simulink model "x11_foc_iden_flux"  (R2023b)
settings: Solver=VariableStepAuto  StartTime=0.0  StopTime=0.5  RelTol=1e-3
values from neighbouring files (symbols this model uses):
  Fcoef = 0    [foc_para.m]
  Flux = 0.00525    [foc_para.m]
  gamma_now = 10*(Flux*Flux)    (= 0.000275625)    [foc_para.m]
  Jx = 0.000004483738    (= 4.483738e-06)    [foc_para.m]
  Ls = 0.00042    [foc_para.m]
  Np = 4    [foc_para.m]
  Rs = 0.45    [foc_para.m]
  Tpwm = 4000-1    (= 3999)    [foc_para.m]
  Ts = 1/SwitchFrequency    (= 5e-05)    [foc_para.m]
  vbus = 24    [foc_para.m]
undefined symbols (not defined in the file or in its folder): DiscIntNeverNeededParam
libraries: spsMosfetLib x6, spsVoltageMeasurementLib x3, simulink x1, spsPermanentMagnetSynchronousMachineLib x1, spsDCVoltageSourceLib x1, spspowerguiLib x1
settings Model: Creator=disnox  LastModifiedBy=disno
settings DataIOCC: ReturnWorkspaceOutputs=off
settings DebuggingCC: ParameterPrecisionLossMsg=none

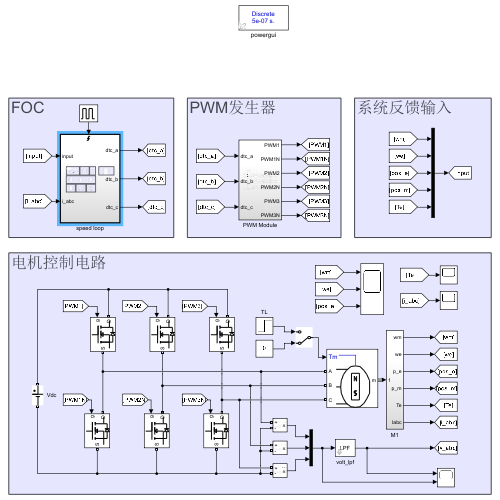
[thumbnail: Simulink's stored preview of the top-level diagram]
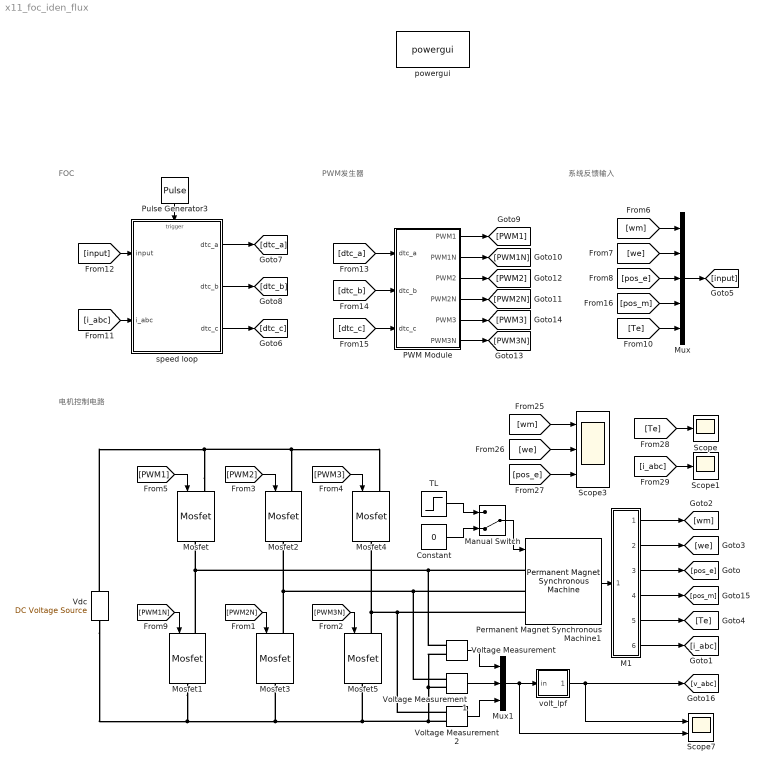
== system x11_foc_iden_flux ==
  note: FOC
  note: PWM发生器
  note: 系统反馈输入
  note: 电机控制电路
  Constant : Constant  Value=0
  M1 : Subsystem
  Manual Switch : ManualSwitch  CurrentSetting=0
  Mosfet{,1..5} (6 alike) : spsMosfetLib/Mosfet  Ron=0.1  Lon=0  Rd=0.01  Vfd=0  IC=0  Rs=1e5  Cs=inf  Measurements=off
  Mux : Mux  Inputs=5
  Mux1 : Mux  Inputs=3
  PWM Module : Subsystem
  Permanent Magnet Synchronous Machine1 : spsPermanentMagnetSynchronousMachineLib/Permanent Magnet Synchronous Machine  NbPhases=3  FluxDistribution=Sinusoidal  RotorType=Salient-pole  MechanicalLoad=Torque Tm  PresetModel=No  ShowDetailedParameters=on  MeasurementBus=off  Resistance=(Rs)  Inductance=8.5e-3  dqInductances=[Ls, Ls]  La=0.000835  MachineConstant=Flux linkage established by magnets (V.s)  Flux=Flux  VoltageCst=3.809  TorqueCst=0.0315  Flat=120  Mechanical=[Jx Fcoef Np 0]  PolePairs=Np  InitialConditions=[0,0, 0,0]  InitialConditions5ph=[0 0 0 0 0 0]  RefAngle=Aligned with phase A axis (original Park)  IterativeDiscreteModel=Trapezoidal non iterative  TsBlock=-1  TsPowergui=0
  Pulse Generator3 : DiscretePulseGenerator  PulseType=Time based  Period=Ts  PulseWidth=50
  Scope : Scope
  Scope1 : Scope
  Scope3 : Scope  NumInputPorts=3
  Scope7 : Scope  NumInputPorts=2
  TL : Step  Time=0.1  After=0.05  SampleTime=0
  Vdc : spsDCVoltageSourceLib/DC Voltage Source  Amplitude=vbus  Measurements=None
  Voltage Measurement : spsVoltageMeasurementLib/Voltage Measurement  PhasorSimulation=off  OutputType=Complex  PSBequivalent=0
  Voltage Measurement1 : spsVoltageMeasurementLib/Voltage Measurement  PhasorSimulation=off  OutputType=Complex  PSBequivalent=0
  Voltage Measurement2 : spsVoltageMeasurementLib/Voltage Measurement  PhasorSimulation=off  OutputType=Complex  PSBequivalent=0
  powergui : spspowerguiLib/powergui  SimulationMode=Discrete  SampleTime=Ts/100  frequency=60  Iterations=50  frequencyindice=0  Pbase=100e6  ErrMax=1e-4  UnitsV=kV  UnitsW=MW  buscounter=0  FunctionMessages=off  echomessages=off  EnableUseOfTLC=off  CurrentSourceSwitches=off  DisableSnubberDevices=off  DisableRonSwitches=off  DisableVfSwitches=off  DisplayEquations=off  AutomaticDiscreteSolvers=off  SolverType=Tustin/Backward Euler (TBE)  Interpol=off  ExternalGateDelay=off  methode=off  Ts=0  x0status=blocks  SPID=off  SwTol=0  HookPort=off  NonlinearTolerance=1e-4  nMaxIteration=100  ContinueOnMaxIteration=off  RestoreLinks=warning  ResistiveCurrentMeasurement=off  Frange=[0:2:500]  Ylog=off  Xlog=on  ShowGrid=off  save=off  variable=ZData  structure=0  ZoomFFT=off  StartTime=0.0  cycles=1  DisplayStyle=1  fundamental=60  FreqAxis=off  MaxFrequency=1000  frequencyindicesteady=1  RmsSteady=1  display=off
  speed loop : Subsystem
  volt_lpf : Subsystem  mask{lpf_freq=1000, Ts=Ts/100}
      mask DialogControl ParameterGroupVar Prompt: 参数
      mask Display: disp('LPF')
  wires:
  Pulse Generator3/1 -> speed loop/Trigger
  [input] -> speed loop/1(input)
  speed loop/2(dtc_b) -> [dtc_b]
  speed loop/1(dtc_a) -> [dtc_a]
  speed loop/3(dtc_c) -> [dtc_c]
  [dtc_a] -> PWM Module/1(dtc_a)
  [dtc_b] -> PWM Module/2(dtc_b)
  [dtc_c] -> PWM Module/3(dtc_c)
  PWM Module/1(PWM1) -> [PWM1]
  PWM Module/2(PWM1N) -> [PWM1N]
  PWM Module/3(PWM2) -> [PWM2]
  PWM Module/4(PWM2N) -> [PWM2N]
  PWM Module/5(PWM3) -> [PWM3]
  PWM Module/6(PWM3N) -> [PWM3N]
  [i_abc] -> speed loop/2(i_abc)
  Mux/1 -> [input]
  [Te] -> Mux/5
  [pos_m] -> Mux/4
  [pos_e] -> Mux/3
  [we] -> Mux/2
  [wm] -> Mux/1
  Mux1/1 -> Scope7/2, volt_lpf/1(in)
  Voltage Measurement/1 -> Mux1/1
  [i_abc] -> Scope1/1
  M1/4(p_m) -> [pos_m]
  Voltage Measurement2/1 -> Mux1/3
  TL/1 -> Manual Switch/1
  M1/1(wm) -> [wm]
  [Te] -> Scope/1
  M1/3(p_e) -> [pos_e]
  Permanent Magnet Synchronous Machine1/1 -> M1/1(In1)
  M1/6(Iabc) -> [i_abc]
  [PWM2] -> Mosfet2/1
  [PWM1N] -> Mosfet1/1
  [PWM3N] -> Mosfet5/1
  [pos_e] -> Scope3/3
  [PWM3] -> Mosfet4/1
  volt_lpf/1(out) -> Scope7/1, [v_abc]
  Manual Switch/1 -> Permanent Magnet Synchronous Machine1/1
  [PWM1] -> Mosfet/1
  [we] -> Scope3/2
  Constant/1 -> Manual Switch/2
  M1/5(Te) -> [Te]
  M1/2(we) -> [we]
  [PWM2N] -> Mosfet3/1
  Voltage Measurement1/1 -> Mux1/2
  [wm] -> Scope3/1
  connections:
  Mosfet3/RConn1 -- Voltage Measurement2/LConn2 -- Voltage Measurement1/LConn2 -- Voltage Measurement/LConn2 -- Mosfet5/RConn1 -- Vdc/LConn1 -- Mosfet1/RConn1
  Mosfet/RConn1 -- Mosfet1/LConn1 -- Permanent Magnet Synchronous Machine1/LConn1 -- Voltage Measurement/LConn1
  Voltage Measurement1/LConn1 -- Mosfet3/LConn1 -- Mosfet2/RConn1 -- Permanent Magnet Synchronous Machine1/LConn2
  Mosfet/LConn1 -- Vdc/RConn1 -- Mosfet2/LConn1 -- Mosfet4/LConn1
  Mosfet4/RConn1 -- Mosfet5/LConn1 -- Permanent Magnet Synchronous Machine1/LConn3 -- Voltage Measurement2/LConn1

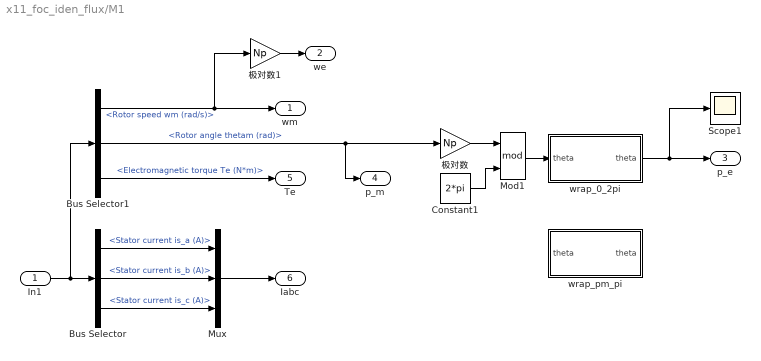
== system x11_foc_iden_flux/M1 ==
  In1 : Inport
  Bus Selector : BusSelector  OutputSignals=Stator current is_a (A),Stator current is_b (A),Stator current is_c (A)
  Bus Selector1 : BusSelector  OutputSignals=Rotor speed wm (rad/s),Rotor angle thetam (rad),Electromagnetic torque Te (N*m)
  Constant1 : Constant  Value=2*pi
  Mod1 : Math  Operator=mod
  Mux : Mux  Inputs=3
  Scope1 : Scope
  wrap_0_2pi : MATLAB Function  TreatAsAtomicUnit=on
  wrap_pm_pi : MATLAB Function  TreatAsAtomicUnit=on
  极对数 : Gain  Gain=Np
  极对数1 : Gain  Gain=Np
  wm : Outport
  we : Outport  Port=2
  p_e : Outport  Port=3
  p_m : Outport  Port=4
  Te : Outport  Port=5
  Iabc : Outport  Port=6
  wires:
  Bus Selector/1 -> Mux/1  "<Stator current is_a (A)>"
  Bus Selector/2 -> Mux/2  "<Stator current is_b (A)>"
  Bus Selector/3 -> Mux/3  "<Stator current is_c (A)>"
  Bus Selector1/1 -> 极对数1/1, wm/1  "<Rotor speed wm (rad/s)>"
  Bus Selector1/2 -> p_m/1, 极对数/1  "<Rotor angle thetam (rad)>"
  Bus Selector1/3 -> Te/1  "<Electromagnetic torque Te (N*m)>"
  Mux/1 -> Iabc/1
  In1/1 -> Bus Selector1/1, Bus Selector/1
  Constant1/1 -> Mod1/2
  极对数/1 -> Mod1/1
  Mod1/1 -> wrap_0_2pi/1("theta ")
  wrap_0_2pi/1(theta) -> Scope1/1, p_e/1
  极对数1/1 -> we/1

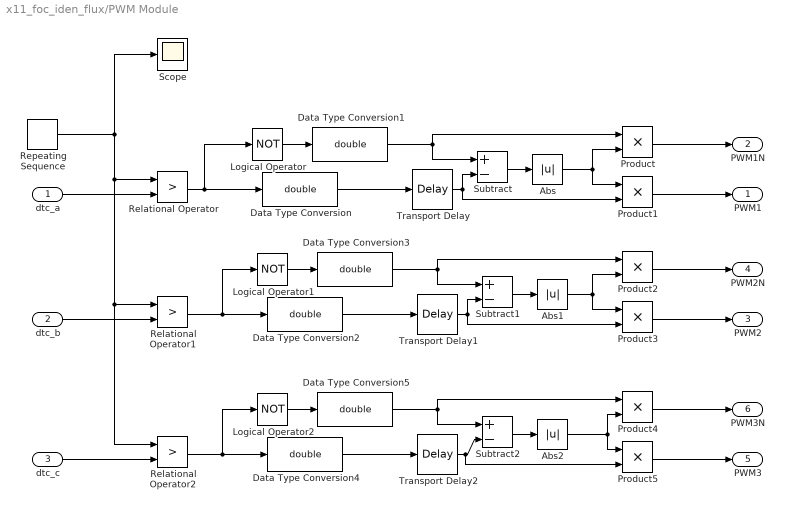
== system x11_foc_iden_flux/PWM Module ==
  dtc_a : Inport
  dtc_b : Inport  Port=2
  dtc_c : Inport  Port=3
  Abs : Abs  SaturateOnIntegerOverflow=off
  Abs1 : Abs  SaturateOnIntegerOverflow=off
  Abs2 : Abs  SaturateOnIntegerOverflow=off
  Data Type Conversion{,1..5} (6 alike) : DataTypeConversion  OutDataTypeStr=double  SaturateOnIntegerOverflow=off  RndMeth=Floor
  Logical Operator : Logic  Operator=NOT  AllPortsSameDT=off  OutDataTypeStr=boolean
  Logical Operator1 : Logic  Operator=NOT  AllPortsSameDT=off  OutDataTypeStr=boolean
  Logical Operator2 : Logic  Operator=NOT  AllPortsSameDT=off  OutDataTypeStr=boolean
  Product{,1..5} (6 alike) : Product
  Relational Operator : RelationalOperator  Operator=>  OutDataTypeStr=boolean  RndMeth=Simplest  InputSameDT=off
  Relational Operator1 : RelationalOperator  Operator=>  OutDataTypeStr=boolean  RndMeth=Simplest  InputSameDT=off
  Relational Operator2 : RelationalOperator  Operator=>  OutDataTypeStr=boolean  RndMeth=Simplest  InputSameDT=off
  Repeating Sequence : simulink/Sources/Repeating Sequence  rep_seq_t=[0 Ts/2 Ts]  rep_seq_y=[0 Tpwm 0]
  Scope : Scope
  Subtract : Sum  Inputs=+-
  Subtract1 : Sum  Inputs=+-
  Subtract2 : Sum  Inputs=+-
  Transport Delay : TransportDelay  DelayTime=168/168e6
  Transport Delay1 : TransportDelay  DelayTime=168/168e6
  Transport Delay2 : TransportDelay  DelayTime=168/168e6
  PWM1 : Outport
  PWM1N : Outport  Port=2
  PWM2 : Outport  Port=3
  PWM2N : Outport  Port=4
  PWM3 : Outport  Port=5
  PWM3N : Outport  Port=6
  wires:
  Product1/1 -> PWM1/1
  Relational Operator1/1 -> Logical Operator1/1, Data Type Conversion2/1
  Logical Operator2/1 -> Data Type Conversion5/1
  Subtract/1 -> Abs/1
  Relational Operator2/1 -> Data Type Conversion4/1, Logical Operator2/1
  Product4/1 -> PWM3N/1
  Data Type Conversion5/1 -> Subtract2/1, Product4/1
  Product2/1 -> PWM2N/1
  Abs1/1 -> Product2/2, Product3/1
  Transport Delay2/1 -> Subtract2/2, Product5/2
  Repeating Sequence/1 -> Scope/1, Relational Operator/1, Relational Operator2/1, Relational Operator1/1
  Data Type Conversion/1 -> Transport Delay/1
  Product/1 -> PWM1N/1
  Product3/1 -> PWM2/1
  Abs2/1 -> Product5/1, Product4/2
  Data Type Conversion2/1 -> Transport Delay1/1
  dtc_a/1 -> Relational Operator/2
  Transport Delay/1 -> Product1/2, Subtract/2
  Subtract1/1 -> Abs1/1
  Data Type Conversion3/1 -> Subtract1/1, Product2/1
  dtc_c/1 -> Relational Operator2/2
  Logical Operator/1 -> Data Type Conversion1/1
  Transport Delay1/1 -> Product3/2, Subtract1/2
  Relational Operator/1 -> Logical Operator/1, Data Type Conversion/1
  Abs/1 -> Product/2, Product1/1
  Product5/1 -> PWM3/1
  Data Type Conversion4/1 -> Transport Delay2/1
  Subtract2/1 -> Abs2/1
  Logical Operator1/1 -> Data Type Conversion3/1
  Data Type Conversion1/1 -> Subtract/1, Product/1
  dtc_b/1 -> Relational Operator1/2

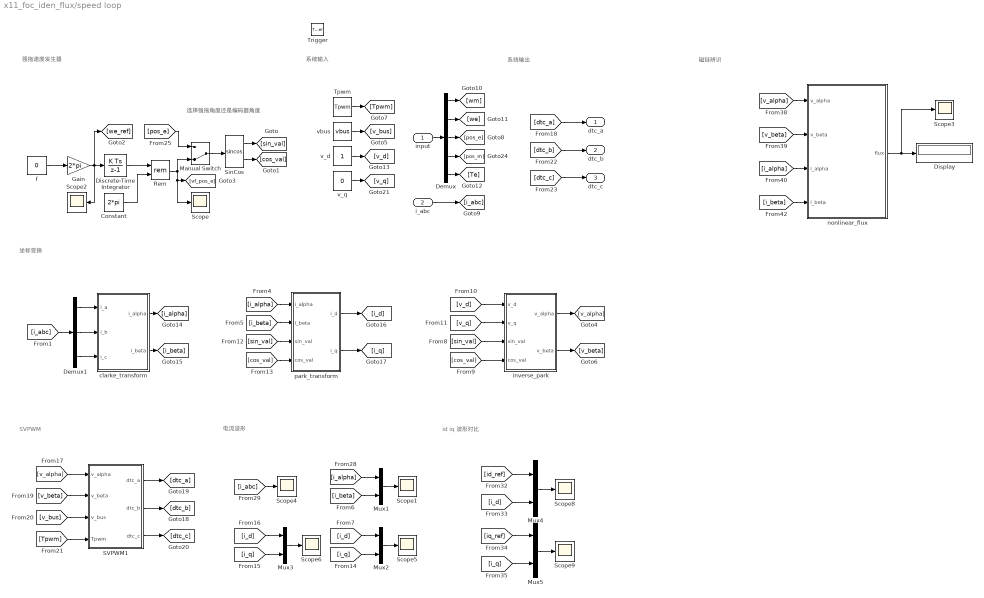
== system x11_foc_iden_flux/speed loop ==
  note: 坐标变换
  note: SVPWM
  note: 电流波形
  note: 系统输入
  note: 系统输出
  note: id iq 波形对比
  note: 磁链辨识
  note: 选择强拖角度还是编码器角度
  note: 强拖速度发生器
  input : Inport
  i_abc : Inport  Port=2
  Trigger : TriggerPort  VariantControl=(inherit)
  Constant : Constant  Value=2*pi
  Demux : Demux  Outputs=5
  Demux1 : Demux  Outputs=3
  Discrete-Time Integrator : DiscreteIntegrator  SampleTime=-1  ICPrevOutput=DiscIntNeverNeededParam  ICPrevScaledInput=DiscIntNeverNeededParam
  Display : Display
  Gain : Gain  Gain=2*pi
  Manual Switch : ManualSwitch  CurrentSetting=0
  Mux{1..5} (5 alike) : Mux  Inputs=2
  Rem : Math  Operator=rem
  SVPWM1 : Subsystem  TreatAsAtomicUnit=on
      settings: RTWSystemCode=Nonreusable function  RTWFcnNameOpts=Use subsystem name
  Scope{,1..6,8..9} (9 alike) : Scope
  SinCos : Trigonometry  Operator=sincos
  Tpwm : Constant  Value=Tpwm
  clarke_transform : Subsystem  TreatAsAtomicUnit=on
      settings: RTWSystemCode=Nonreusable function  RTWFcnNameOpts=Use subsystem name
  f : Constant  Value=0
  inverse_park : Subsystem  TreatAsAtomicUnit=on
      settings: RTWSystemCode=Nonreusable function  RTWFcnNameOpts=Use subsystem name
  nonlinear_flux : Subsystem  TreatAsAtomicUnit=on
      settings: RTWSystemCode=Nonreusable function  RTWFcnNameOpts=Use subsystem name
  park_transform : Subsystem  TreatAsAtomicUnit=on
      settings: RTWSystemCode=Nonreusable function  RTWFcnNameOpts=Use subsystem name
  v_d : Constant
  v_q : Constant  Value=0
  vbus : Constant  Value=vbus
  dtc_a : Outport
  dtc_b : Outport  Port=2
  dtc_c : Outport  Port=3
  wires:
  [cos_val] -> inverse_park/4(cos_val)
  [sin_val] -> park_transform/3(sin_val)
  [v_d] -> inverse_park/1(v_d)
  [v_q] -> inverse_park/2(v_q)
  [cos_val] -> park_transform/4(cos_val)
  [sin_val] -> inverse_park/3(sin_val)
  [v_beta] -> SVPWM1/2(v_beta)
  [v_alpha] -> SVPWM1/1(v_alpha)
  [Tpwm] -> SVPWM1/4(Tpwm)
  [v_bus] -> SVPWM1/3(v_bus)
  Tpwm/1 -> [Tpwm]
  vbus/1 -> [v_bus]
  inverse_park/2(v_beta) -> [v_beta]
  inverse_park/1(v_alpha) -> [v_alpha]
  Demux1/1 -> clarke_transform/1(i_a)
  Demux1/2 -> clarke_transform/2(i_b)
  Demux1/3 -> clarke_transform/3(i_c)
  [i_abc] -> Demux1/1
  i_abc/1 -> [i_abc]
  [i_alpha] -> park_transform/1(i_alpha)
  [i_beta] -> park_transform/2(i_beta)
  clarke_transform/1(i_alpha) -> [i_alpha]
  clarke_transform/2(i_beta) -> [i_beta]
  park_transform/1(i_d) -> [i_d]
  park_transform/2(i_q) -> [i_q]
  [i_abc] -> Scope4/1
  [i_alpha] -> Mux1/1
  Mux1/1 -> Scope1/1
  [i_beta] -> Mux1/2
  [i_q] -> Mux2/2
  [i_d] -> Mux2/1
  Mux2/1 -> Scope5/1
  [i_d] -> Mux3/1
  Mux3/1 -> Scope6/1
  [i_q] -> Mux3/2
  [dtc_b] -> dtc_b/1
  [dtc_c] -> dtc_c/1
  [dtc_a] -> dtc_a/1
  SVPWM1/3(dtc_c) -> [dtc_c]
  SVPWM1/2(dtc_b) -> [dtc_b]
  SVPWM1/1(dtc_a) -> [dtc_a]
  [id_ref] -> Mux4/1
  Mux4/1 -> Scope8/1
  [i_d] -> Mux4/2
  [iq_ref] -> Mux5/1
  Mux5/1 -> Scope9/1
  [i_q] -> Mux5/2
  Demux/3 -> [pos_e]
  Demux/5 -> [Te]
  Demux/2 -> [we]
  Demux/4 -> [pos_m]
  input/1 -> Demux/1
  Demux/1 -> [wm]
  [v_alpha] -> nonlinear_flux/1(v_alpha)
  [v_beta] -> nonlinear_flux/2(v_beta)
  [i_alpha] -> nonlinear_flux/3(i_alpha)
  [i_beta] -> nonlinear_flux/4(i_beta)
  v_d/1 -> [v_d]
  v_q/1 -> [v_q]
  Rem/1 -> Scope/1, [vf_pos_e], Manual Switch/2
  f/1 -> Gain/1
  Constant/1 -> Rem/2
  Discrete-Time Integrator/1 -> Rem/1
  SinCos/1 -> [sin_val]
  SinCos/2 -> [cos_val]
  Manual Switch/1 -> SinCos/1
  [pos_e] -> Manual Switch/1
  Gain/1 -> [we_ref], Scope2/1, Discrete-Time Integrator/1
  nonlinear_flux/1(flux) -> Scope3/1, Display/1

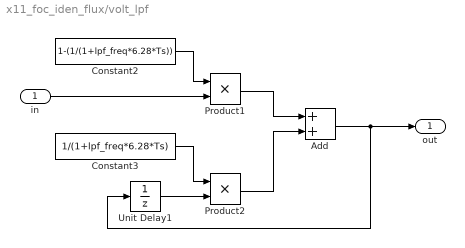
== system x11_foc_iden_flux/volt_lpf ==
  in : Inport
  Add : Sum
  Constant2 : Constant  Value=1-(1/(1+lpf_freq*6.28*Ts))
  Constant3 : Constant  Value=1/(1+lpf_freq*6.28*Ts)
  Product1 : Product
  Product2 : Product
  Unit Delay1 : UnitDelay  SampleTime=-1  HasFrameUpgradeWarning=on
  out : Outport
  wires:
  Constant3/1 -> Product2/1
  Constant2/1 -> Product1/1
  Product1/1 -> Add/1
  Unit Delay1/1 -> Product2/2
  Add/1 -> out/1, Unit Delay1/1
  Product2/1 -> Add/2
  in/1 -> Product1/2

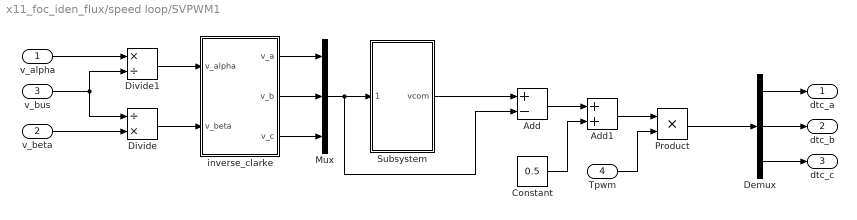
== system x11_foc_iden_flux/speed loop/SVPWM1 ==
  v_alpha : Inport
  v_beta : Inport  Port=2
  v_bus : Inport  Port=3
  Tpwm : Inport  Port=4
  Add : Sum  Inputs=+-
  Add1 : Sum
  Constant : Constant  Value=0.5
  Demux : Demux  Outputs=3
  Divide : Product  Inputs=/*
  Divide1 : Product  Inputs=*/
  Mux : Mux  Inputs=3
  Product : Product
  Subsystem : Subsystem
  inverse_clarke : Subsystem  TreatAsAtomicUnit=on
      settings: RTWSystemCode=Nonreusable function  RTWFcnNameOpts=Use subsystem name
  dtc_a : Outport
  dtc_b : Outport  Port=2
  dtc_c : Outport  Port=3
  wires:
  Demux/1 -> dtc_a/1
  Demux/2 -> dtc_b/1
  Demux/3 -> dtc_c/1
  inverse_clarke/2(v_b) -> Mux/2
  inverse_clarke/1(v_a) -> Mux/1
  inverse_clarke/3(v_c) -> Mux/3
  Mux/1 -> Subsystem/1(v_abc), Add/2
  Subsystem/1(vcom) -> Add/1
  Add/1 -> Add1/1
  Constant/1 -> Add1/2
  Add1/1 -> Product/1
  Product/1 -> Demux/1
  Tpwm/1 -> Product/2
  Divide/1 -> inverse_clarke/2(v_beta)
  Divide1/1 -> inverse_clarke/1(v_alpha)
  v_alpha/1 -> Divide1/1
  v_beta/1 -> Divide/2
  v_bus/1 -> Divide/1, Divide1/2

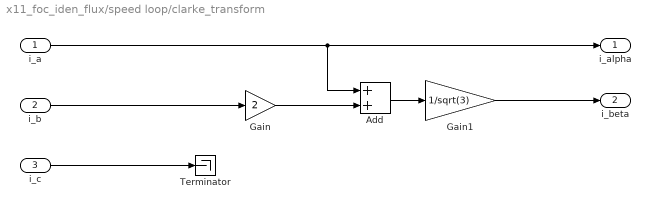
== system x11_foc_iden_flux/speed loop/clarke_transform ==
  i_a : Inport
  i_b : Inport  Port=2
  i_c : Inport  Port=3
  Add : Sum
  Gain : Gain  Gain=2
  Gain1 : Gain  Gain=1/sqrt(3)
  Terminator : Terminator
  i_alpha : Outport
  i_beta : Outport  Port=2
  wires:
  i_a/1 -> Add/1, i_alpha/1
  i_b/1 -> Gain/1
  Gain/1 -> Add/2
  Add/1 -> Gain1/1
  Gain1/1 -> i_beta/1
  i_c/1 -> Terminator/1

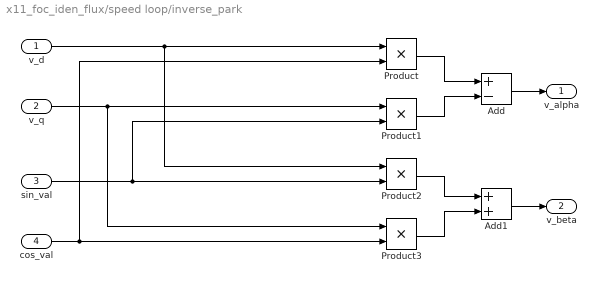
== system x11_foc_iden_flux/speed loop/inverse_park ==
  v_d : Inport
  v_q : Inport  Port=2
  sin_val : Inport  Port=3
  cos_val : Inport  Port=4
  Add : Sum  Inputs=+-
  Add1 : Sum  AccumDataTypeStr=double
  Product{,1..3} (4 alike) : Product
  v_alpha : Outport
  v_beta : Outport  Port=2
  wires:
  v_d/1 -> Product2/1, Product/1
  cos_val/1 -> Product3/2, Product/2
  Product/1 -> Add/1
  Product1/1 -> Add/2
  v_q/1 -> Product1/1, Product3/1
  sin_val/1 -> Product2/2, Product1/2
  Add/1 -> v_alpha/1
  Product2/1 -> Add1/1
  Product3/1 -> Add1/2
  Add1/1 -> v_beta/1

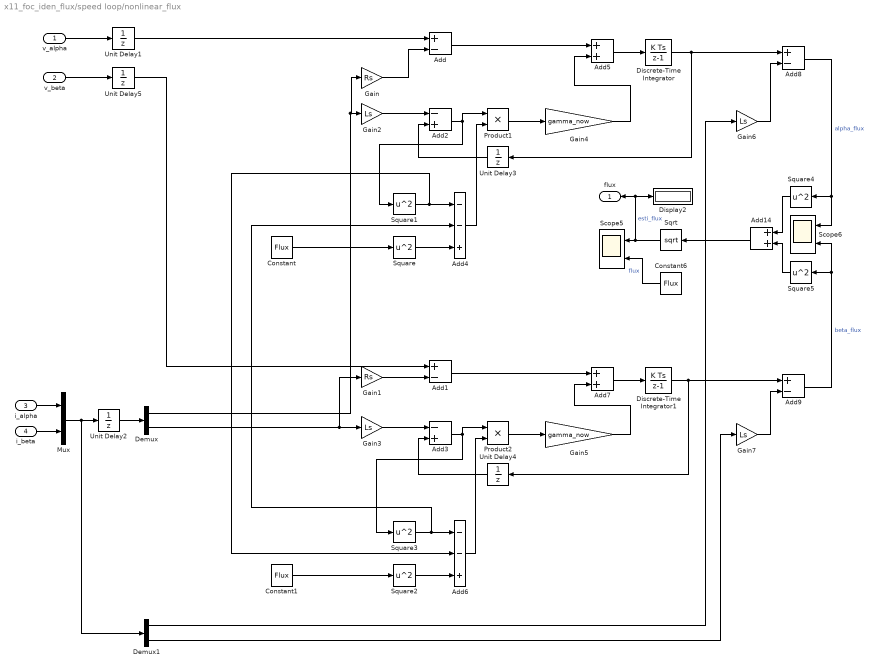
== system x11_foc_iden_flux/speed loop/nonlinear_flux ==
  v_alpha : Inport
  v_beta : Inport  Port=2
  i_alpha : Inport  Port=3
  i_beta : Inport  Port=4
  Add{,1,8..9} (4 alike) : Sum  Inputs=+-
  Add14 : Sum
  Add2 : Sum  Inputs=-+
  Add3 : Sum  Inputs=-+
  Add4 : Sum  Inputs=--+
  Add5 : Sum
  Add6 : Sum  Inputs=--+
  Add7 : Sum
  Constant : Constant  Value=Flux
  Constant1 : Constant  Value=Flux
  Constant6 : Constant  Value=Flux
  Demux : Demux  Outputs=2
  Demux1 : Demux  Outputs=2
  Discrete-Time Integrator : DiscreteIntegrator  InitialCondition=Flux  SampleTime=-1  ICPrevOutput=DiscIntNeverNeededParam  ICPrevScaledInput=DiscIntNeverNeededParam
  Discrete-Time Integrator1 : DiscreteIntegrator  SampleTime=-1  ICPrevOutput=DiscIntNeverNeededParam  ICPrevScaledInput=DiscIntNeverNeededParam
  Display2 : Display
  Gain : Gain  Gain=Rs
  Gain1 : Gain  Gain=Rs
  Gain{2..3,6..7} (4 alike) : Gain  Gain=Ls
  Gain4 : Gain  Gain=gamma_now
  Gain5 : Gain  Gain=gamma_now
  Mux : Mux  Inputs=2
  Product1 : Product
  Product2 : Product
  Scope5 : Scope  NumInputPorts=2
  Scope6 : Scope  NumInputPorts=2
  Sqrt : Sqrt
  Square{,1..5} (6 alike) : Math  Operator=square
  Unit Delay{1..5} (5 alike) : UnitDelay  SampleTime=-1  HasFrameUpgradeWarning=on
  flux : Outport
  wires:
  v_alpha/1 -> Unit Delay1/1
  v_beta/1 -> Unit Delay5/1
  Unit Delay1/1 -> Add/1
  Gain/1 -> Add/2
  i_alpha/1 -> Mux/1
  i_beta/1 -> Mux/2
  Mux/1 -> Unit Delay2/1, Demux1/1
  Unit Delay2/1 -> Demux/1
  Demux/1 -> Gain/1, Gain2/1
  Demux/2 -> Gain3/1, Gain1/1
  Gain1/1 -> Add1/2
  Unit Delay5/1 -> Add1/1
  Gain3/1 -> Add3/1
  Gain2/1 -> Add2/1
  Square/1 -> Add4/3
  Constant/1 -> Square/1
  Add/1 -> Add5/1
  Add2/1 -> Product1/1, Square1/1
  Product1/1 -> Gain4/1
  Unit Delay3/1 -> Add2/2
  Add5/1 -> Discrete-Time Integrator/1
  Gain4/1 -> Add5/2
  Discrete-Time Integrator/1 -> Add8/1, Unit Delay3/1
  Square1/1 -> Add6/2, Add4/1
  Square2/1 -> Add6/3
  Constant1/1 -> Square2/1
  Square3/1 -> Add4/2, Add6/1
  Add7/1 -> Discrete-Time Integrator1/1
  Add1/1 -> Add7/1
  Gain5/1 -> Add7/2
  Product2/1 -> Gain5/1
  Add3/1 -> Product2/1, Square3/1
  Add6/1 -> Product2/2
  Add4/1 -> Product1/2
  Discrete-Time Integrator1/1 -> Add9/1, Unit Delay4/1
  Unit Delay4/1 -> Add3/2
  Demux1/2 -> Gain7/1
  Demux1/1 -> Gain6/1
  Gain7/1 -> Add9/2
  Gain6/1 -> Add8/2
  Add9/1 -> Scope6/2, Square5/1  "beta_flux"
  Add8/1 -> Scope6/1, Square4/1  "alpha_flux"
  Add14/1 -> Sqrt/1
  Sqrt/1 -> flux/1, Display2/1, Scope5/1  "esti_flux"
  Constant6/1 -> Scope5/2  "flux"
  Square5/1 -> Add14/2
  Square4/1 -> Add14/1

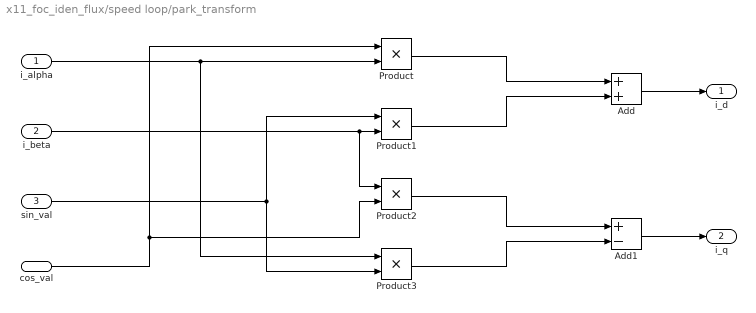
== system x11_foc_iden_flux/speed loop/park_transform ==
  i_alpha : Inport
  i_beta : Inport  Port=2
  sin_val : Inport  Port=3
  cos_val : Inport  Port=4
  Add : Sum
  Add1 : Sum  Inputs=+-
  Product{,1..3} (4 alike) : Product
  i_d : Outport
  i_q : Outport  Port=2
  wires:
  i_alpha/1 -> Product/2, Product3/1
  cos_val/1 -> Product2/2, Product/1
  sin_val/1 -> Product3/2, Product1/1
  i_beta/1 -> Product2/1, Product1/2
  Product/1 -> Add/1
  Product1/1 -> Add/2
  Add/1 -> i_d/1
  Product2/1 -> Add1/1
  Product3/1 -> Add1/2
  Add1/1 -> i_q/1

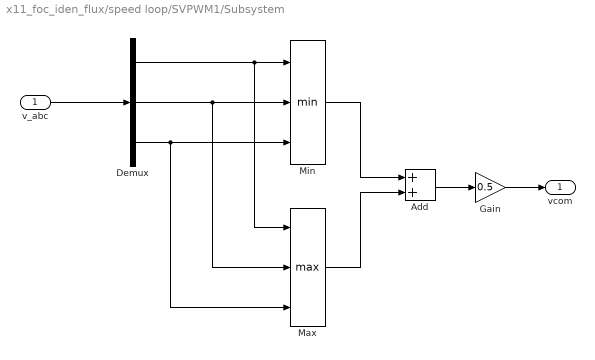
== system x11_foc_iden_flux/speed loop/SVPWM1/Subsystem ==
  v_abc : Inport
  Add : Sum
  Demux : Demux  Outputs=3
  Gain : Gain  Gain=0.5
  Max : MinMax  Function=max  Inputs=3
  Min : MinMax  Inputs=3
  vcom : Outport
  wires:
  Min/1 -> Add/1
  Max/1 -> Add/2
  Add/1 -> Gain/1
  Gain/1 -> vcom/1
  Demux/1 -> Max/1, Min/1
  Demux/2 -> Max/2, Min/2
  Demux/3 -> Max/3, Min/3
  v_abc/1 -> Demux/1

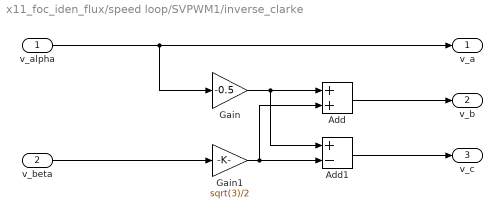
== system x11_foc_iden_flux/speed loop/SVPWM1/inverse_clarke ==
  v_alpha : Inport
  v_beta : Inport  Port=2
  Add : Sum
  Add1 : Sum  Inputs=+-
  Gain : Gain  Gain=-0.5
  Gain1 : Gain  Gain=sqrt(3)/2
  v_a : Outport
  v_b : Outport  Port=2
  v_c : Outport  Port=3
  wires:
  v_alpha/1 -> Gain/1, v_a/1
  Gain/1 -> Add1/1, Add/1
  v_beta/1 -> Gain1/1
  Gain1/1 -> Add/2, Add1/2
  Add/1 -> v_b/1
  Add1/1 -> v_c/1

== matlab function x11_foc_iden_flux/M1/wrap_pm_pi ==
  data: theta output; theta input
function theta = wrap_pm_pi(theta)

    M_PI = pi;
    M_2PI = 2*pi;
    
    if theta > M_PI
        theta = theta - M_2PI;
    elseif theta < -M_PI
        theta = theta + M_2PI;
    end
end

== matlab function x11_foc_iden_flux/M1/wrap_0_2pi ==
  data: theta output; theta input
function theta = wrap_0_2pi(theta)

    M_2PI = 2*pi;
    
    if theta > M_2PI
        theta = theta - M_2PI;
    elseif theta < 0
        theta = theta + M_2PI;
    end
end
